simulink model "Ejercicio_2_DB"  (R2023a)
settings: Solver=VariableStepAuto  StartTime=0.0  StopTime=2  RelTol=1e-6  EnableMultiTasking=on
values from neighbouring files (symbols this model uses):
  Ap = [-Ra/La 0 0 -Kb*A2/(La*R*A1) ... (first row only)    [Ejercicio_1.m]    (also in Ejercicio_2y3.m = [0 1 0)
  b0 = A*A1*R*Kt/(A2*La*JT)    (= 0.0665070497473)    [Ejercicio_2y3.m]
  Bp = [A/La 0 0 0]'    [Ejercicio_1.m]    (also in Ejercicio_2y3.m = [0 0 1]')
  C_DB = eye(3)    [Ejercicio_2y3.m]
  D_DB = [0;0;0]    [Ejercicio_2y3.m]
  g0 = y_inf/(Cp*inv(Bp*Ke-Ap)*Bp)    [Ejercicio_2y3.m]
  Ke = acker(Ap,Bp,P_LC)    [Ejercicio_2y3.m]
settings Model: Creator=54115  LastModifiedBy=franc
settings SolverCC: AlgebraicLoopSolver=TrustRegion
settings DataIOCC: ReturnWorkspaceOutputs=off
settings OptimizationCC: LifeSpan=inf
settings DebuggingCC: UnconnectedInputMsg=warning  UnconnectedOutputMsg=warning  UnconnectedLineMsg=warning  SFUnexpectedBacktrackingDiag=warning  SFNoUnconditionalDefaultTransitionDiag=warning  ArithmeticOperatorsInVariantConditions=warning
settings ModelReferenceCC: EnableRefExpFcnMdlSchedulingChecks=on
settings SFSimCC: SimUseLocalCustomCode=off  CustomCodeUndefinedFunction=UseInterfaceOnly
settings RTWCC: RTWUseLocalCustomCode=off
settings CodeAppCC: StateflowObjectComments=on
settings GRTTargetCC: TargetLangStandard=C89/C90 (ANSI)
settings ConfigComp: CovMetricSettings=dw  CovSaveCumulativeToWorkspaceVar=on  CovSaveSingleToWorkspaceVar=on  CovExternalEMLEnable=off

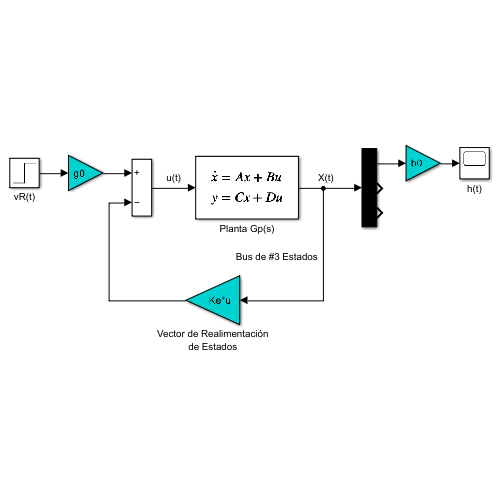
[thumbnail: Simulink's stored preview of the top-level diagram]
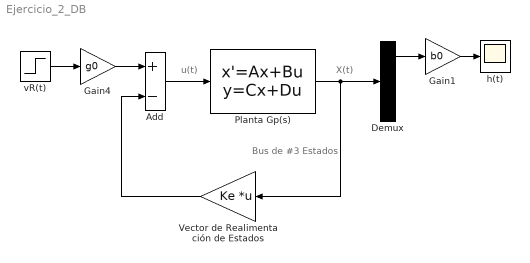
== system Ejercicio_2_DB ==
  note: Bus de #3 Estados
  note: u(t)
  note: X(t)
  Add : Sum  Inputs=+-
  Demux : Demux  Outputs=3
  Gain1 : Gain  Gain=b0
  Gain4 : Gain  Gain=g0
  Planta Gp(s) : StateSpace  A=Ap  B=Bp  C=C_DB  D=D_DB  InitialCondition=0
  Vector de Realimentación de Estados : Gain  Gain=Ke  Multiplication=Matrix(K*u)
  h(t) : Scope
  vR(t) : Step  Time=0  SampleTime=0
  wires:
  Add/1 -> Planta Gp(s)/1
  vR(t)/1 -> Gain4/1
  Planta Gp(s)/1 -> Demux/1, Vector de Realimentación de Estados/1
  Vector de Realimentación de Estados/1 -> Add/2
  Gain4/1 -> Add/1
  Demux/1 -> Gain1/1
  Gain1/1 -> h(t)/1
